simulink model "LocalMaxima_HardThreshold"  (R2020a)
settings: Solver=VariableStepAuto  StartTime=0  StopTime=180  RelTol=1e-3
model workspace (MAT data in the model file):
  a = 0
values from neighbouring files (symbols this model uses):
  fs = 30000    [run_AdaptiveThreshold.m]    (also in run_AdaptiveThresholdLocalMaxima.m; run_HardThreshold.m; run_HardThresholdLocalMaxima.m; run_LocalMaxima_AdaptiveThreshold.m)
  refractory = 10^-3    (= 0.001)    [run_AdaptiveThreshold.m]    (also in run_AdaptiveThresholdLocalMaxima.m; run_HardThreshold.m; run_HardThresholdLocalMaxima.m; run_LocalMaxima_AdaptiveThreshold.m)
  th = [-10]    [run_HardThreshold.m]    (also in run_HardThresholdLocalMaxima.m = [-10:-10:-40]; run_LocalMaxima_HardThreshold.m = [-10:-1:-60]; run_Sample_HardThreshold.m)
libraries: dspfdesign x2, simulink x2, dspswit3 x1, hdlsllib x1
settings Model: SimulationMode=rapid-accelerator  Creator=sbuccelli  LastModifiedBy=diflo

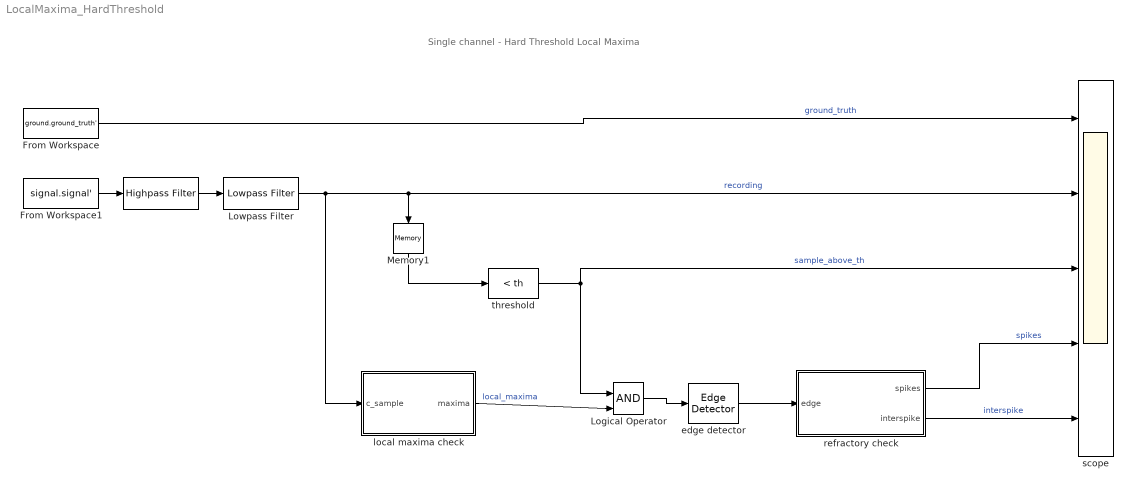
== system LocalMaxima_HardThreshold ==
  note: Single channel - Hard Threshold Local Maxima
  " " : dspfdesign/Highpass Filter  FilterType=IIR  DesignForMinimumOrder=on  FilterOrder=50  StopbandFrequency=1  PassbandFrequency=300  StopbandAttenuation=80  PassbandRipple=0.1  InheritSampleRate=off  SampleRate=fs  SimulateUsing=Interpreted execution  roundingMode=Floor  coeffsDataTypeStr=fixdt(1,16)
  From Workspace : FromWorkspace  VariableName=ground.ground_truth'  SampleTime=1/fs
  From Workspace1 : FromWorkspace  VariableName=signal.signal'  SampleTime=1/fs
  Logical Operator : Logic  IconShape=distinctive  AllPortsSameDT=off  OutDataTypeStr=boolean
  Lowpass Filter : dspfdesign/Lowpass Filter  FilterType=IIR  DesignForMinimumOrder=on  FilterOrder=3  PassbandFrequency=3500  StopbandFrequency=8500  PassbandRipple=0.1  StopbandAttenuation=80  InheritSampleRate=off  SampleRate=fs  SimulateUsing=Interpreted execution  roundingMode=Floor  coeffsDataTypeStr=fixdt(1,16)
  Memory1 : Memory  InheritSampleTime=on
  edge detector : dspswit3/Edge Detector  InputProcessing=Columns as channels (frame based)
      settings: SourceProductBaseCode=DS
  local maxima check : Subsystem
  refractory check : Subsystem
  scope : Scope  NumInputPorts=5
  threshold : simulink/Logic and Bit Operations/Compare To Constant  relop=<  const=th  OutDataTypeStr=boolean
  wires:
  refractory check/1(spikes) -> scope/4  "spikes"
  refractory check/2(interspike) -> scope/5  "interspike"
  edge detector/1 -> refractory check/1("edge ")
  threshold/1 -> Logical Operator/1, scope/3  "sample_above_th"
  Logical Operator/1 -> edge detector/1
  local maxima check/1(maxima) -> Logical Operator/2  "local_maxima"
  Memory1/1 -> threshold/1
  Lowpass Filter/1 -> local maxima check/1(c_sample), scope/2, Memory1/1  "recording"
  From Workspace1/1 -> " "/1
  " "/1 -> Lowpass Filter/1
  From Workspace/1 -> scope/1  "ground_truth"

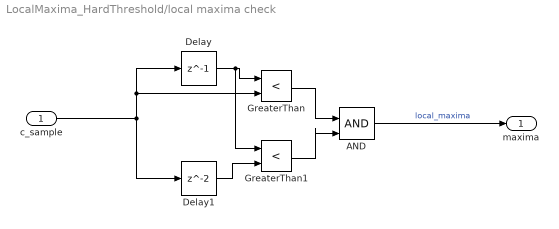
== system LocalMaxima_HardThreshold/local maxima check ==
  c_sample : Inport
  AND : Logic  IconShape=distinctive  AllPortsSameDT=off  OutDataTypeStr=boolean
  Delay : Delay  DelayLength=1  SampleTime=1/30000
  Delay1 : Delay  SampleTime=1/30000
  GreaterThan : RelationalOperator  Operator=<  OutDataTypeStr=boolean  RndMeth=Simplest
  GreaterThan1 : RelationalOperator  Operator=<  OutDataTypeStr=boolean  RndMeth=Simplest
  maxima : Outport
  wires:
  Delay/1 -> GreaterThan1/1, GreaterThan/1
  c_sample/1 -> Delay/1, GreaterThan/2, Delay1/1
  GreaterThan/1 -> AND/1
  GreaterThan1/1 -> AND/2
  AND/1 -> maxima/1  "local_maxima"
  Delay1/1 -> GreaterThan1/2

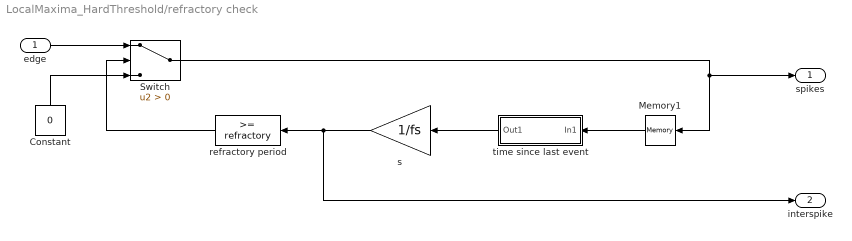
== system LocalMaxima_HardThreshold/refractory check ==
  "edge " : Inport
  Constant : Constant  Value=0
  Memory1 : Memory  InheritSampleTime=on
  Switch : Switch  Criteria=u2 > Threshold
  refractory period : simulink/Logic and Bit Operations/Compare To Constant  relop=>=  const=refractory  OutDataTypeStr=boolean
  s : Gain  Gain=1/fs  ParamDataTypeStr=double
  time since last event : Subsystem
  spikes : Outport
  interspike : Outport  Port=2
  wires:
  "edge "/1 -> Switch/1
  Memory1/1 -> time since last event/1(In1)
  time since last event/1(Out1) -> s/1
  Constant/1 -> Switch/3
  s/1 -> refractory period/1, interspike/1
  Switch/1 -> spikes/1, Memory1/1
  refractory period/1 -> Switch/2

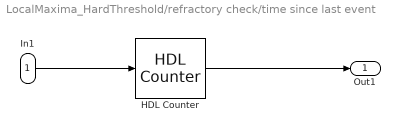
== system LocalMaxima_HardThreshold/refractory check/time since last event ==
  In1 : Inport
  HDL Counter : hdlsllib/Sources/HDL Counter  CountType=Free running  CountInit=1  CountStep=1  CountMax=25  CountFromType=Initial value  CountFrom=1  CountResetPort=on  CountLoadPort=off  CountEnbPort=off  CountDirPort=off  CountDataType=Unsigned  CountWordLen=32  CountFracLen=0  CountSampTime=1
  Out1 : Outport
  wires:
  In1/1 -> HDL Counter/1
  HDL Counter/1 -> Out1/1
